simulink model "Sterowanie_Statkiem"  (Simulink 10.0)
settings: Solver=FixedStepAuto  StartTime=0.0  StopTime=10  FixedStep=0.001  MaxStep=0.01  MinStep=0.001  RelTol=1e-3
settings Model: Creator=szymo  LastModifiedBy=szymo
settings DataIOCC: SaveFormat=Dataset  ReturnWorkspaceOutputs=on
settings OptimizationCC: LifeSpan=auto
settings DebuggingCC: UnderspecifiedInitializationDetection=Simplified  MergeDetectMultiDrivingBlocksExec=error  SFUnexpectedBacktrackingDiag=error  SFNoUnconditionalDefaultTransitionDiag=error  SFExecutionAtInitializationDiag=warning  UnderSpecifiedDimensionMsg=warning  ArithmeticOperatorsInVariantConditions=error
settings HardwareCC: ProdBitPerPointer=64  ProdBitPerSizeT=64  ProdBitPerPtrDiffT=64  ProdLargestAtomicFloat=Float  ProdIntDivRoundTo=Zero  ProdEndianess=LittleEndian  ProdWordSize=64  ProdHWDeviceType=Intel->x86-64 (Windows64)
settings ModelReferenceCC: PropagateSignalLabelsOutOfModel=on
settings SFSimCC: SimUseLocalCustomCode=on  CustomCodeUndefinedFunction=FilterOut
settings RTWCC: RTWUseLocalCustomCode=on
settings CodeAppCC: StateflowObjectComments=off
settings GRTTargetCC: TargetLangStandard=C99 (ISO)  CombineOutputUpdateFcns=on  GRTInterface=off
settings ConfigComp: CovMetricSettings=dwe  CovHtmlReporting=off  CovSaveCumulativeToWorkspaceVar=off  CovSaveSingleToWorkspaceVar=off

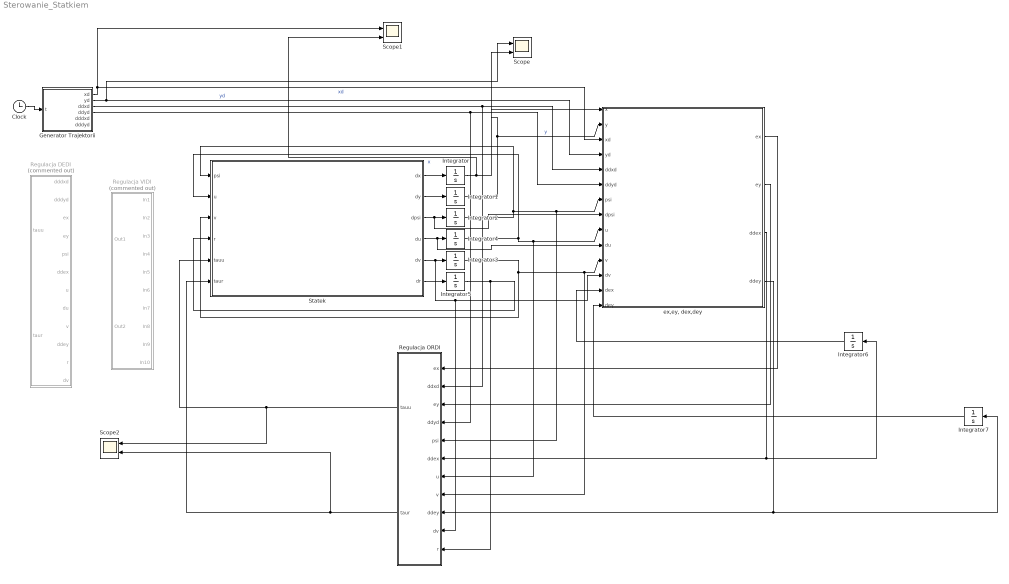
== system Sterowanie_Statkiem ==
  Clock : Clock
  Generator Trajektorii : MATLAB Function  TreatAsAtomicUnit=on
  Integrator : Integrator  InitialCondition=-0.01
  Integrator1 : Integrator  InitialCondition=1.01
  Integrator2 : Integrator  InitialCondition=0.01
  Integrator3 : Integrator  InitialCondition=0.1
  Integrator4 : Integrator  InitialCondition=.1
  Integrator5 : Integrator  InitialCondition=0.1
  Integrator6 : Integrator
  Integrator7 : Integrator
  Regulacja DEDI : Subsystem  Commented=on
  Regulacja ORDI : Subsystem
  Regulacja VIDI : Subsystem  Commented=on
  Scope : Scope  NumInputPorts=2
  Scope1 : Scope  NumInputPorts=2
  Scope2 : Scope  NumInputPorts=2
  Statek : MATLAB Function  TreatAsAtomicUnit=on
  "ex,ey, dex,dey" : MATLAB Function  TreatAsAtomicUnit=on
  wires:
  Statek/1(dx) -> Integrator/1
  Statek/2(dy) -> Integrator1/1
  Statek/3(dpsi) -> "ex,ey, dex,dey"/8(dpsi), Integrator2/1
  Integrator/1 -> Scope1/2, "ex,ey, dex,dey"/1(x)  "x"
  Integrator1/1 -> Scope/2, "ex,ey, dex,dey"/2(y)  "y"
  Statek/4(du) -> "ex,ey, dex,dey"/10(du), Integrator4/1
  Statek/5(dv) -> Regulacja ORDI/10(dv), "ex,ey, dex,dey"/12(dv), Integrator3/1
  Statek/6(dr) -> Integrator5/1
  Integrator2/1 -> Statek/1(psi), Regulacja ORDI/5(psi), "ex,ey, dex,dey"/7(psi)
  Integrator4/1 -> Regulacja ORDI/7(u), "ex,ey, dex,dey"/9(u), Statek/2(u)
  Integrator3/1 -> Statek/3(v), Regulacja ORDI/8(v), "ex,ey, dex,dey"/11(v)
  Integrator5/1 -> Regulacja ORDI/11(r), Statek/4(r)
  Clock/1 -> Generator Trajektorii/1(t)
  Generator Trajektorii/1(xd) -> Scope1/1, "ex,ey, dex,dey"/3(xd)  "xd"
  Generator Trajektorii/2(yd) -> Scope/1, "ex,ey, dex,dey"/4(yd)  "yd"
  Generator Trajektorii/3(ddxd) -> Regulacja ORDI/2(ddxd), "ex,ey, dex,dey"/5(ddxd)
  Generator Trajektorii/4(ddyd) -> Regulacja ORDI/4(ddyd), "ex,ey, dex,dey"/6(ddyd)
  Regulacja ORDI/1(tauu) -> Scope2/1, Statek/5(tauu)
  Regulacja ORDI/2(taur) -> Scope2/2, Statek/6(taur)
  "ex,ey, dex,dey"/1(ex) -> Regulacja ORDI/1(ex)
  "ex,ey, dex,dey"/2(ey) -> Regulacja ORDI/3(ey)
  "ex,ey, dex,dey"/4(ddey) -> Regulacja ORDI/9(ddey), Integrator7/1
  "ex,ey, dex,dey"/3(ddex) -> Regulacja ORDI/6(ddex), Integrator6/1
  Integrator7/1 -> "ex,ey, dex,dey"/14(dey)
  Integrator6/1 -> "ex,ey, dex,dey"/13(dex)

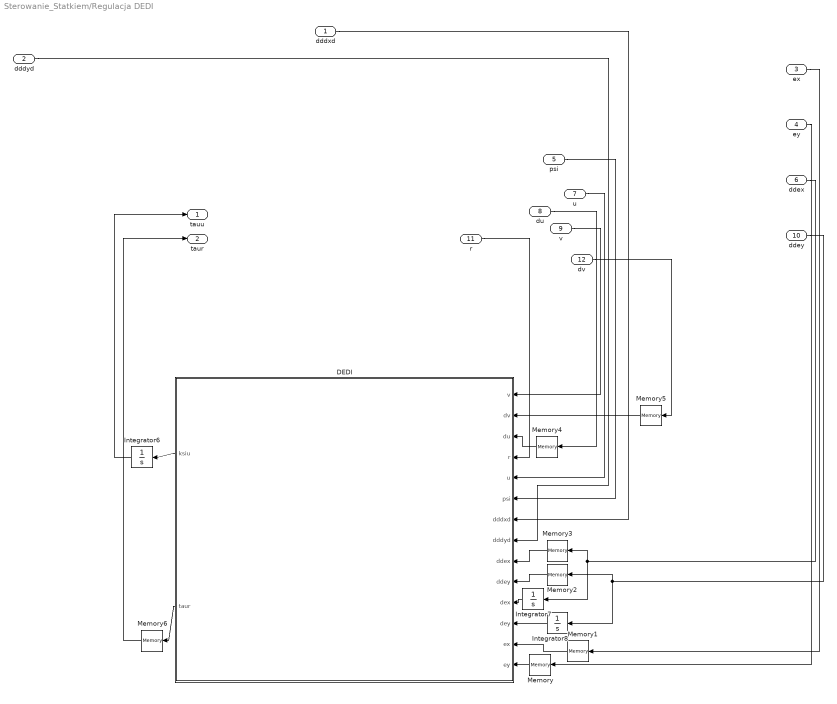
== system Sterowanie_Statkiem/Regulacja DEDI ==
  dddxd : Inport
  dddyd : Inport  Port=2
  ex : Inport  Port=3
  ey : Inport  Port=4
  psi : Inport  Port=5
  ddex : Inport  Port=6
  u : Inport  Port=7
  du : Inport  Port=8
  v : Inport  Port=9
  ddey : Inport  Port=10
  r : Inport  Port=11
  dv : Inport  Port=12
  DEDI : MATLAB Function  TreatAsAtomicUnit=on
  Integrator6 : Integrator
  Integrator7 : Integrator
  Integrator8 : Integrator
  Memory{,1..6} (7 alike) : Memory
  tauu : Outport
  taur : Outport  Port=2
  wires:
  ddey/1 -> Memory2/1, Integrator8/1
  Memory2/1 -> DEDI/10(ddey)
  DEDI/1(ksiu) -> Integrator6/1
  DEDI/2(taur) -> Memory6/1
  Memory6/1 -> taur/1
  Memory1/1 -> DEDI/13(ex)
  ey/1 -> Memory/1
  Integrator7/1 -> DEDI/11(dex)
  Integrator8/1 -> DEDI/12(dey)
  ddex/1 -> Integrator7/1, Memory3/1
  Memory3/1 -> DEDI/9(ddex)
  Memory4/1 -> DEDI/3(du)
  Memory5/1 -> DEDI/2(dv)
  ex/1 -> Memory1/1
  Memory/1 -> DEDI/14(ey)
  u/1 -> DEDI/5(u)
  du/1 -> Memory4/1
  psi/1 -> DEDI/6(psi)
  Integrator6/1 -> tauu/1
  r/1 -> DEDI/4(r)
  dddxd/1 -> DEDI/7(dddxd)
  dddyd/1 -> DEDI/8(dddyd)
  dv/1 -> Memory5/1
  v/1 -> DEDI/1(v)

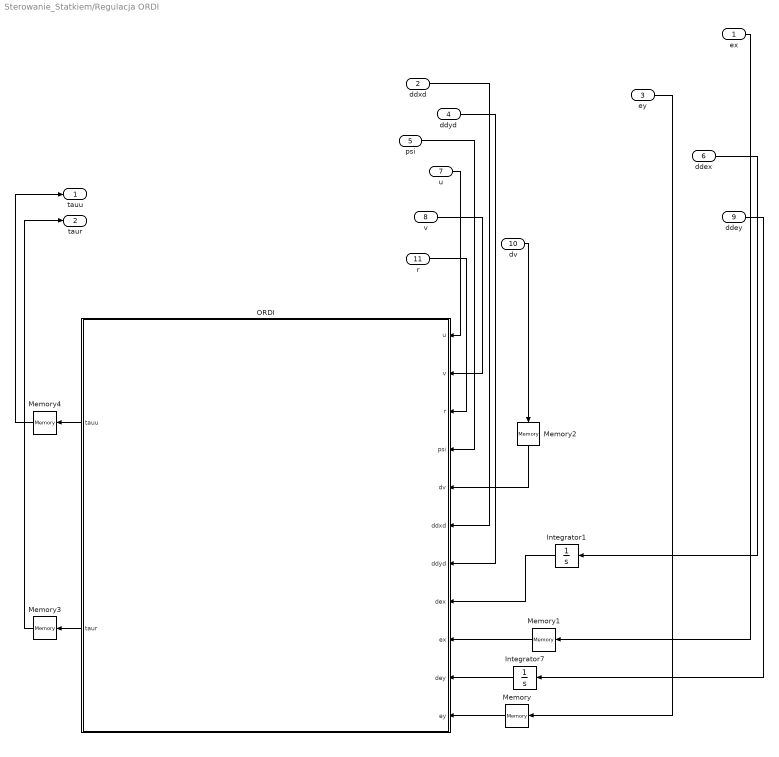
== system Sterowanie_Statkiem/Regulacja ORDI ==
  ex : Inport
  ddxd : Inport  Port=2
  ey : Inport  Port=3
  ddyd : Inport  Port=4
  psi : Inport  Port=5
  ddex : Inport  Port=6
  u : Inport  Port=7
  v : Inport  Port=8
  ddey : Inport  Port=9
  dv : Inport  Port=10
  r : Inport  Port=11
  Integrator1 : Integrator
  Integrator7 : Integrator
  Memory{,1..4} (5 alike) : Memory
  ORDI : MATLAB Function  TreatAsAtomicUnit=on
  tauu : Outport
  taur : Outport  Port=2
  wires:
  ddey/1 -> Integrator7/1
  ORDI/2(taur) -> Memory3/1
  Integrator7/1 -> ORDI/10(dey)
  Memory2/1 -> ORDI/5(dv)
  Memory/1 -> ORDI/11(ey)
  r/1 -> ORDI/3(r)
  ORDI/1(tauu) -> Memory4/1
  v/1 -> ORDI/2(v)
  Memory1/1 -> ORDI/9(ex)
  u/1 -> ORDI/1(u)
  psi/1 -> ORDI/4(psi)
  dv/1 -> Memory2/1
  Memory3/1 -> taur/1
  ey/1 -> Memory/1
  ddyd/1 -> ORDI/7(ddyd)
  ddxd/1 -> ORDI/6(ddxd)
  Memory4/1 -> tauu/1
  ex/1 -> Memory1/1
  ddex/1 -> Integrator1/1
  Integrator1/1 -> ORDI/8(dex)

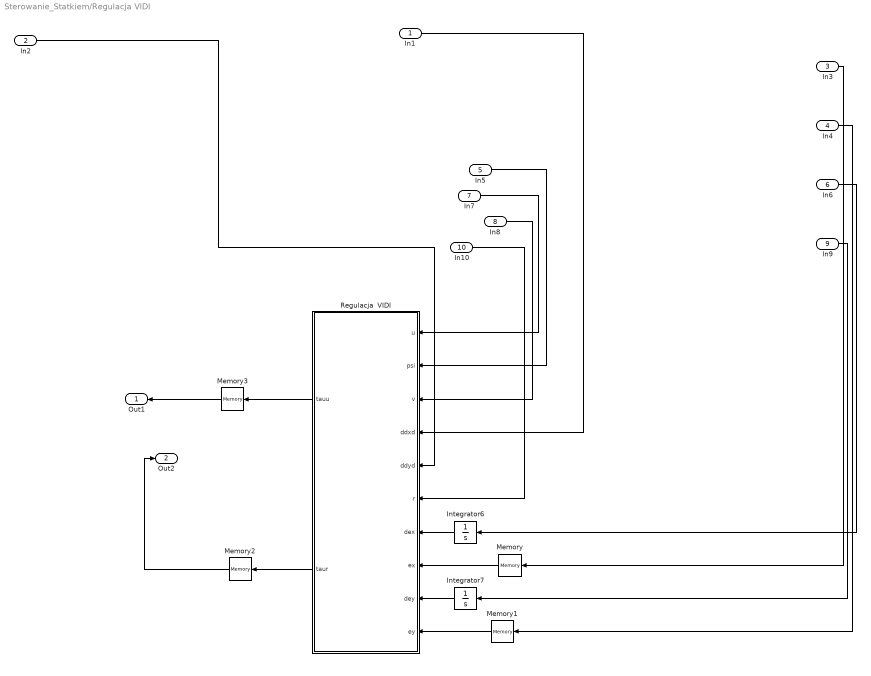
== system Sterowanie_Statkiem/Regulacja VIDI ==
  In1 : Inport
  In2 : Inport  Port=2
  In3 : Inport  Port=3
  In4 : Inport  Port=4
  In5 : Inport  Port=5
  In6 : Inport  Port=6
  In7 : Inport  Port=7
  In8 : Inport  Port=8
  In9 : Inport  Port=9
  In10 : Inport  Port=10
  Integrator6 : Integrator
  Integrator7 : Integrator
  Memory{,1..3} (4 alike) : Memory
  Regulacja  VIDI : MATLAB Function  TreatAsAtomicUnit=on
  Out1 : Outport
  Out2 : Outport  Port=2
  wires:
  Memory1/1 -> Regulacja  VIDI/10(ey)
  In9/1 -> Integrator7/1
  In2/1 -> Regulacja  VIDI/5(ddyd)
  Integrator6/1 -> Regulacja  VIDI/7(dex)
  In1/1 -> Regulacja  VIDI/4(ddxd)
  Regulacja  VIDI/1(tauu) -> Memory3/1
  Memory/1 -> Regulacja  VIDI/8(ex)
  Integrator7/1 -> Regulacja  VIDI/9(dey)
  In8/1 -> Regulacja  VIDI/3(v)
  Regulacja  VIDI/2(taur) -> Memory2/1
  Memory2/1 -> Out2/1
  In5/1 -> Regulacja  VIDI/2(psi)
  In10/1 -> Regulacja  VIDI/6(r)
  In6/1 -> Integrator6/1
  In7/1 -> Regulacja  VIDI/1(u)
  In4/1 -> Memory1/1
  In3/1 -> Memory/1
  Memory3/1 -> Out1/1

== matlab function Generator Trajektorii ==
  data: t input double; xd output double; yd output double; ddxd output double; ddyd output double; dddxd output double; dddyd output double
function [xd,yd,ddxd,ddyd,dddxd,dddyd] = fcn(t)

xd = sin(t);
yd = cos(t);
ddxd = -sin(t);
ddyd = -cos(t);
dddxd = -cos(t);
dddyd = sin(t);

== matlab function Statek ==
  data: psi input double size=1; u input double size=1; v input double size=1; dx output double size=1; r input double size=1; dy output double size=1; dpsi output double size=1; du output double size=1; dv output double size=1; dr output double size=1; tauu input double size=1; taur input double size=1
function [dx,dy,dpsi,du,dv,dr] = fcn(psi,u,v,r,tauu,taur)
m11=1.956;
m22=2.405;
m33=0.043;
d11=2.436;
d22=12.992;
d33=0.0564;
dx = u*cos(psi)-v*sin(psi);
dy = u*sin(psi)+v*cos(psi);
dpsi = r;
du = (m22*v*r-d11*u+tauu)/m11;
dv = (-m11*u*r-d22*v)/m22;
dr = ((m11-m22)*u*v-d33*r+taur)/m33;

== matlab function ex,ey, dex,dey ==
  data: x input double; y input double; xd input double; yd input double; ddxd input double; ddyd input double; psi input double; dpsi input double; u input double; du input double; v input double; dv input double; ex output double; ey output double; ddex output double; ddey output double; dex input double; dey input double
function [ex,ey,ddex,ddey] = fcn(x,y,xd,yd,ddxd,ddyd,psi,dpsi,u,du,v,dv,dex,dey)

ex = x-xd;
ey = y-yd;

%% NOWE
m11=1.956;
m22=2.405;
m33=0.043;
d11=2.436;
d22=12.992;
d33=0.0564;
k31=4;
k32=4;
k33=4;
k34=4;
l=0.01;

%ddex = -k31*dex-k32*ex;
%ddey = -k33*dey-k34*ey;

%%
ddex = du*cos(psi)-u*dpsi*sin(psi)-dv*sin(psi)-v*dpsi*cos(psi)-ddxd;
ddey = du*sin(psi)+u*dpsi*cos(psi)+dv*cos(psi)-v*dpsi*sin(psi)-ddyd;

== matlab function Regulacja DEDI/DEDI ==
  data: v input double; dv input double; du input double; r input double; u input double; ksiu output double; psi input double; dddxd input double; dddyd input double; ddex input double; ddey input double; dex input double; dey input double; ex input double; ey input double; taur output double
function [ksiu,taur] = fcn(v,dv,du,r,u,psi,dddxd,dddyd,ddex,ddey,dex,dey,ex,ey)

m11=1.956;
m22=2.405;
m33=0.043;
d11=2.436;
d22=12.992;
d33=0.0564;

k11=6;
k12=12;
k13=8;
k14=6;
k15=12;
k16=8;

%fu = (m22*v*r-d11*u)/m11;
fr = ((m11-m22)*u*v-d33*r)/m33;
%gu = 1/m11;
%gr = 1/m33;

au = (m22*dv*r+m22*v*fr-d11*du)/m11;
av = (-m11*du*r-m11*u*fr-d22*dv)/m22;
%bu = m22*v/(m11*m33);
%bv = -m11*u/(m22*m33);

F1 = [(au-2*dv*r-v*fr-u*r^2)*cos(psi)-(av+2*du*r+u*fr-v*r^2)*sin(psi)-dddxd; (au-2*dv*r-v*fr-u*r^2)*sin(psi)+(av+2*du*r+u*fr-v*r^2)*cos(psi)-dddyd];
G1 = [cos(psi)/m11, ((m22/m11-1)*v*cos(psi)+(m11/m22-1)*u*sin(psi))/m33; sin(psi)/m11, ((m22/m11-1)*v*sin(psi)+(1-m11/m22)*u*cos(psi))/m33];


wek = G1^(-1)*(-1*F1+[-k11*ddex-k12*dex-k13*ex;-k14*ddey-k15*dey-k16*ey]);
ksiu = wek(1);
taur = wek(2);

== matlab function Regulacja VIDI/Regulacja  VIDI ==
  data: u input double; tauu output double; psi input double; v input double; ddxd input double; ddyd input double; r input double; dex input double; ex input double; dey input double; ey input double; taur output double
function [tauu, taur] = fcn(u,psi,v,ddxd,ddyd,r,dex,ex,dey,ey)
k21=4; %pogorszyl
k22=4; %ten na 10, reszta na 1 daje dobrego x
k23=4; %pogorszyl
k24=4; %przyblizyl y ale nie tak szybko
k25=2;% blad symulacji
lambda=10;
m11=1.956;
m22=2.405;
m33=0.043;
d11=2.436;
d22=12.992;
d33=0.0564;

fr = ((m11-m22)*u*v-d33*r)/m33;
gr = 1/m33;

G2 = [cos(psi)/m11 m22*v*cos(psi)/m11+m11*u*sin(psi)/m22-u*sin(psi)-v*cos(psi); sin(psi)/m11 m22*v*sin(psi)/m11-m11*u*cos(psi)/m22+u*cos(psi)-v*sin(psi)];
F2 = [-d11*u*cos(psi)/m11+d22*v*sin(psi)*m22-ddxd; -d11*u*sin(psi)/m11-d22*v*cos(psi)/m22-ddyd];
wek = (G2)^(-1)*(-1*F2+[-k21*dex-k22*ex;-k23*dey-k24*ey]);
tauu = wek(1);
rd = wek(2);
taur = gr^(-1)*(lambda*(rd-r)-fr-k25*(rd-r));

== matlab function Regulacja ORDI/ORDI ==
  data: u input double; tauu output double; v input double; r input double; psi input double; dv input double; ddxd input double; ddyd input double; dex input double; ex input double; dey input double; ey input double; taur output double
function [tauu,taur] = fcn(u,v,r,psi,dv,ddxd,ddyd,dex,ex,dey,ey)
m11=1.956;
m22=2.405;
m33=0.043;
d11=2.436;
d22=12.992;
d33=0.0564;
k31=4;
k32=4;
k33=4;
k34=4;
l=0.01;

fu = (m22*v*r-d11*u)/m11;
fr = ((m11-m22)*u*v-d33*r)/m33;
F = [fu*cos(psi)-u*r*sin(psi)-dv*sin(psi)-v*r*cos(psi)-ddxd;fu*sin(psi)+u*r*cos(psi)+dv*cos(psi)-v*r*sin(psi)-ddyd];
F3 = F + [-l*fr*sin(psi) - l*r^2*cos(psi);l*fr*cos(psi)-l*r^2*sin(psi)];
G3 = [cos(psi)/m11 -l*sin(psi)/m33; sin(psi)/m11 l*cos(psi)/m33];
wek = (G3)^(-1)*(-1*F3+[-k31*dex-k32*ex; -k33*dey - k34*ey]);
tauu = wek(1);
taur = wek(2);
